simulink model "MPC_constrained"  (R2024a)
settings: Solver=VariableStepAuto  StartTime=0.0  StopTime=1  RelTol=1e-3
values from neighbouring files (symbols this model uses):
  N = 5    [project_script.m]    (also in scriptpoint7.m)
  N3 = 100    [project_script.m]    (also in scriptpoint7.m)
  Qd = 1*eye(2)    [project_script.m]    (also in scriptpoint7.m = 1000*eye(2))
  Rd = 1*eye(2)    [project_script.m]    (also in scriptpoint7.m)
  S0 = zeros(2)    [project_script.m]    (also in scriptpoint7.m)
  Ts = 1/8000    (= 0.000125)    [project_script.m]    (also in scriptpoint7.m)
  u_bar_d = Bd\ (eye(size(Ad))-Ad)*xref    [project_script.m]    (also in scriptpoint7.m)
  u_sat_max = [u1_max; u2_max]    [project_script.m]    (also in scriptpoint7.m)
  u_sat_min = [u1_min; u2_min]    [project_script.m]    (also in scriptpoint7.m)
  x0 = [x0_1;x0_2]    [project_script.m]    (also in scriptpoint7.m)
  x_sat_max = [x1_max; x2_max]    [project_script.m]    (also in scriptpoint7.m)
  x_sat_min = [x1_min; x2_min]    [project_script.m]    (also in scriptpoint7.m)
  xref = [6.9; 8.9]    [project_script.m]    (also in scriptpoint7.m)
undefined symbols (not defined in the file or in its folder): Ad, Bd, Cd, Dd, Kd, mympc, Qd2, Rd2, Sd, Sd2
settings Model: Creator=Utente  LastModifiedBy=Utente

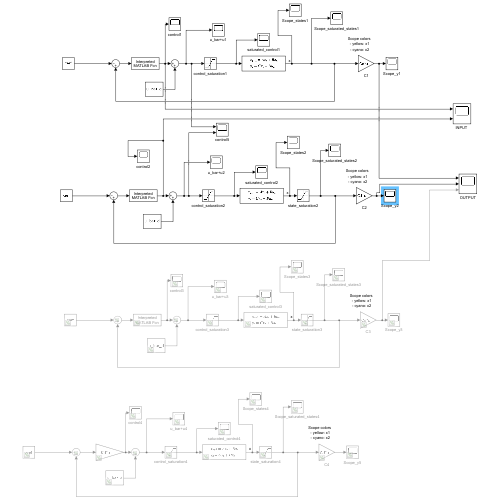
[thumbnail: Simulink's stored preview of the top-level diagram]
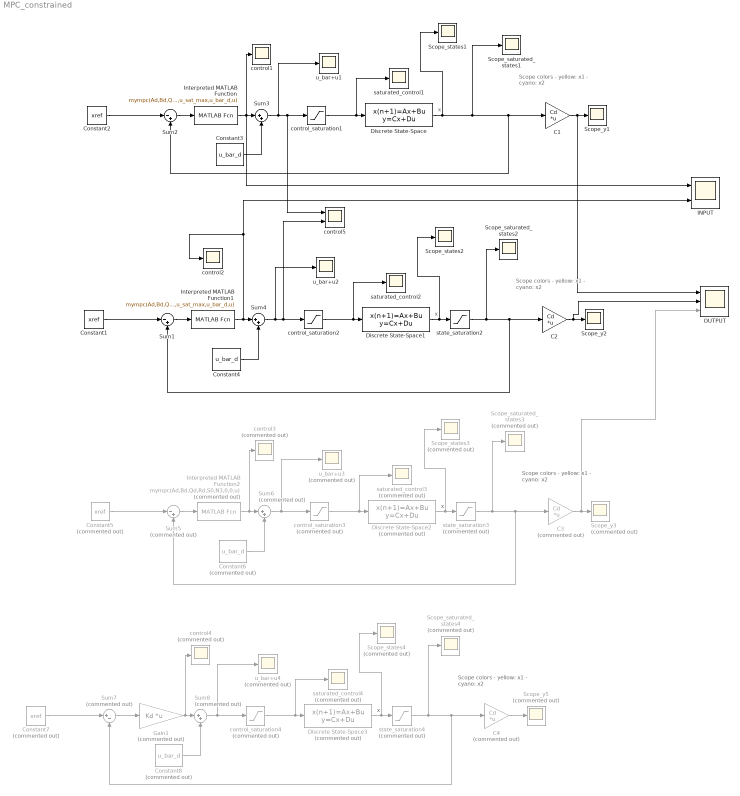
== system MPC_constrained ==
  note: x
  note: Scope colors
      | - yellow: x1
      | - cyano: x2
  note: x
  note: Scope colors
      | - yellow: x1
      | - cyano: x2
  note: x
  note: Scope colors
      | - yellow: x1
      | - cyano: x2
  note: x
  note: Scope colors
      | - yellow: x1
      | - cyano: x2
  C1 : Gain  Gain=Cd  Multiplication=Matrix(K*u)
  C2 : Gain  Gain=Cd  Multiplication=Matrix(K*u)
  C3 : Gain  Commented=on  Gain=Cd  Multiplication=Matrix(K*u)
  C4 : Gain  Commented=on  Gain=Cd  Multiplication=Matrix(K*u)
  Constant1 : Constant  Value=xref  SampleTime=Ts
  Constant2 : Constant  Value=xref  SampleTime=Ts
  Constant3 : Constant  Value=u_bar_d  SampleTime=Ts
  Constant4 : Constant  Value=u_bar_d  SampleTime=Ts
  Constant5 : Constant  Commented=on  Value=xref  SampleTime=Ts
  Constant6 : Constant  Commented=on  Value=u_bar_d  SampleTime=Ts
  Constant7 : Constant  Commented=on  Value=xref  SampleTime=Ts
  Constant8 : Constant  Commented=on  Value=u_bar_d  SampleTime=Ts
  Discrete State-Space : DiscreteStateSpace  A=Ad  B=Bd  C=Cd  D=Dd  InitialCondition=x0  SampleTime=Ts
  Discrete State-Space1 : DiscreteStateSpace  A=Ad  B=Bd  C=Cd  D=Dd  InitialCondition=x0  SampleTime=Ts
  Discrete State-Space2 : DiscreteStateSpace  Commented=on  A=Ad  B=Bd  C=Cd  D=Dd  InitialCondition=x0  SampleTime=Ts
  Discrete State-Space3 : DiscreteStateSpace  Commented=on  A=Ad  B=Bd  C=Cd  D=Dd  InitialCondition=x0  SampleTime=Ts
  Gain1 : Gain  Commented=on  Gain=Kd  Multiplication=Matrix(K*u)
  "INPUT " : Scope  NumInputPorts=2
  Interpreted MATLAB Function : MATLABFcn  MATLABFcn=mympc(Ad,Bd,Qd,Rd,Sd,N,u_sat_min,u_sat_max,u_bar_d,u)
  Interpreted MATLAB Function1 : MATLABFcn  MATLABFcn=mympc(Ad,Bd,Qd2,Rd2,Sd2,N,u_sat_min,u_sat_max,u_bar_d,u)
  Interpreted MATLAB Function2 : MATLABFcn  Commented=on  MATLABFcn=mympc(Ad,Bd,Qd,Rd,S0,N3,0,0,u)
  OUTPUT : Scope  NumInputPorts=3
  Scope_saturated_states1 : Scope
  Scope_saturated_states2 : Scope
  Scope_saturated_states3 : Scope  Commented=on
  Scope_saturated_states4 : Scope  Commented=on
  Scope_states1 : Scope
  Scope_states2 : Scope
  Scope_states3 : Scope  Commented=on
  Scope_states4 : Scope  Commented=on
  Scope_y1 : Scope
  Scope_y2 : Scope
  Scope_y3 : Scope  Commented=on
  Scope_y5 : Scope  Commented=on
  Sum1 : Sum  Inputs=|-+
  Sum2 : Sum  Inputs=|-+
  Sum3 : Sum  Inputs=|++
  Sum4 : Sum  Inputs=|++
  Sum5 : Sum  Commented=on  Inputs=|-+
  Sum6 : Sum  Commented=on  Inputs=|++
  Sum7 : Sum  Commented=on  Inputs=|+-
  Sum8 : Sum  Commented=on  Inputs=|++
  control1 : Scope
  control2 : Scope
  control3 : Scope  Commented=on
  control4 : Scope  Commented=on
  control5 : Scope  NumInputPorts=2
  control_saturation1 : Saturate  UpperLimit=u_sat_max  LowerLimit=u_sat_min
  control_saturation2 : Saturate  UpperLimit=u_sat_max  LowerLimit=u_sat_min
  control_saturation3 : Saturate  Commented=on  UpperLimit=u_sat_max  LowerLimit=u_sat_min
  control_saturation4 : Saturate  Commented=on  UpperLimit=u_sat_max  LowerLimit=u_sat_min
  saturated_control1 : Scope
  saturated_control2 : Scope
  saturated_control3 : Scope  Commented=on
  saturated_control4 : Scope  Commented=on
  state_saturation2 : Saturate  UpperLimit=x_sat_max  LowerLimit=x_sat_min
  state_saturation3 : Saturate  Commented=on  UpperLimit=x_sat_max  LowerLimit=x_sat_min
  state_saturation4 : Saturate  Commented=on  UpperLimit=x_sat_max  LowerLimit=x_sat_min
  u_bar+u1 : Scope
  u_bar+u2 : Scope
  u_bar+u3 : Scope  Commented=on
  u_bar+u4 : Scope  Commented=on
  wires:
  Sum3/1 -> control5/1, control_saturation1/1, u_bar+u1/1
  control_saturation1/1 -> saturated_control1/1, Discrete State-Space/1
  C1/1 -> OUTPUT/1, Scope_y1/1
  Constant2/1 -> Sum2/1
  Discrete State-Space/1 -> Sum2/2, C1/1, Scope_saturated_states1/1, Scope_states1/1
  Constant3/1 -> Sum3/2
  Sum2/1 -> Interpreted MATLAB Function/1
  Interpreted MATLAB Function/1 -> "INPUT "/1, control1/1, Sum3/1
  Sum1/1 -> Interpreted MATLAB Function1/1
  Interpreted MATLAB Function1/1 -> "INPUT "/2, control2/1, Sum4/1
  Constant4/1 -> Sum4/2
  state_saturation2/1 -> Sum1/2, C2/1, Scope_saturated_states2/1
  Constant1/1 -> Sum1/1
  Sum4/1 -> control5/2, control_saturation2/1, u_bar+u2/1
  control_saturation2/1 -> saturated_control2/1, Discrete State-Space1/1
  Discrete State-Space1/1 -> Scope_states2/1, state_saturation2/1
  C2/1 -> OUTPUT/2, Scope_y2/1
  Sum5/1 -> Interpreted MATLAB Function2/1
  Interpreted MATLAB Function2/1 -> control3/1, Sum6/1
  Constant6/1 -> Sum6/2
  state_saturation3/1 -> Sum5/2, C3/1, Scope_saturated_states3/1
  Constant5/1 -> Sum5/1
  Sum6/1 -> control_saturation3/1, u_bar+u3/1
  control_saturation3/1 -> saturated_control3/1, Discrete State-Space2/1
  Discrete State-Space2/1 -> Scope_states3/1, state_saturation3/1
  C3/1 -> OUTPUT/3, Scope_y3/1
  Constant7/1 -> Sum7/1
  control_saturation4/1 -> saturated_control4/1, Discrete State-Space3/1
  Constant8/1 -> Sum8/2
  C4/1 -> Scope_y5/1
  Sum8/1 -> control_saturation4/1, u_bar+u4/1
  state_saturation4/1 -> Sum7/2, C4/1, Scope_saturated_states4/1
  Gain1/1 -> control4/1, Sum8/1
  Discrete State-Space3/1 -> Scope_states4/1, state_saturation4/1
  Sum7/1 -> Gain1/1
